simulink subsystem "Piero"  (R2023b)
settings: Solver=VariableStepAuto  StartTime=0.0  StopTime=10.0  RelTol=1e-3
settings Model: Creator=juana  LastModifiedBy=juana

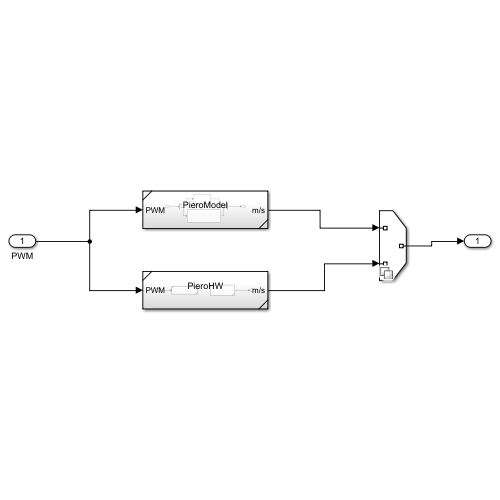
[thumbnail: Simulink's stored preview of the top-level diagram]
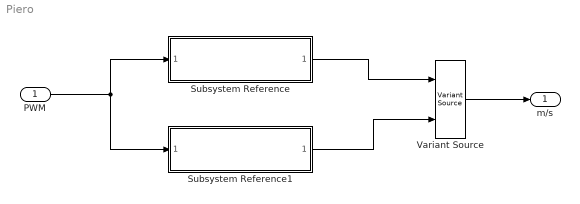
== system Piero ==
  PWM : Inport  OutMin=[-255]  OutMax=[255]
  Subsystem Reference : Subsystem  ReferencedSubsystem=PieroModel
  Subsystem Reference1 : Subsystem  ReferencedSubsystem=PieroHW
  Variant Source : VariantSource
  m/s : Outport
  wires:
  Variant Source/1 -> m/s/1
  Subsystem Reference/1 -> Variant Source/1
  Subsystem Reference1/1 -> Variant Source/2
  PWM/1 -> Subsystem Reference1/1, Subsystem Reference/1
